simulink model "Verification_Actuator_Primitive"  (R2012b)
settings: Solver=FixedStepDiscrete  StartTime=0.0  StopTime=10.0  FixedStep=0.1  RelTol=1e-3
libraries: sldvlib x7
settings Model: Creator=Kerianne  LastModifiedBy=Kerianne
settings DataIOCC: SaveFormat=Structure
settings OptimizationCC: InlineParams=on

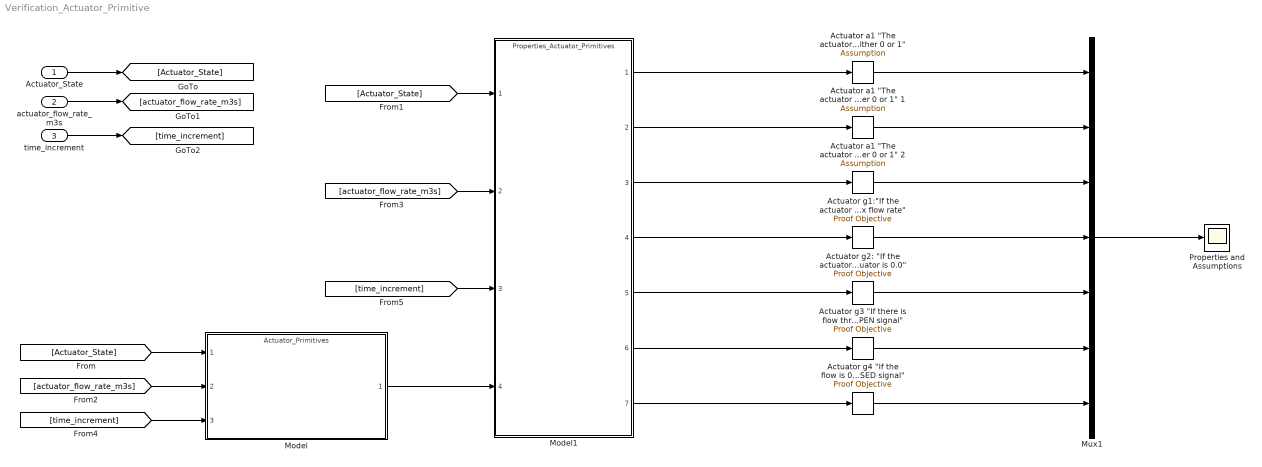
== system Verification_Actuator_Primitive ==
  Actuator_State : Inport  OutDataTypeStr=double
  actuator_flow_rate_m3s : Inport  Port=2  OutDataTypeStr=double
  time_increment : Inport  Port=3  OutDataTypeStr=double
  "Actuator a1 \"The actuator state is either 0 or 1\" " : sldvlib/Objectives and Constraints/Assumption  enabled=on  customAVTBlockType=Assumption  intervals=true  initial=off  dispValues=on  outEnabled=on
      settings: AttributesFormatString=%<intervals>
  "Actuator a1 \"The actuator state is either 0 or 1\" 1" : sldvlib/Objectives and Constraints/Assumption  enabled=on  customAVTBlockType=Assumption  intervals=true  initial=off  dispValues=on  outEnabled=on
      settings: AttributesFormatString=%<intervals>
  "Actuator a1 \"The actuator state is either 0 or 1\" 2" : sldvlib/Objectives and Constraints/Assumption  enabled=on  customAVTBlockType=Assumption  intervals=true  initial=off  dispValues=on  outEnabled=on
      settings: AttributesFormatString=%<intervals>
  "Actuator g1:\"If the actuator is receiving an ON|OPEN signal then the flow through the actuator is the max flow rate\"" : sldvlib/Objectives and Constraints/Proof Objective  enabled=on  customAVTBlockType=Proof Objective  intervals=true  dispValues=on  outEnabled=on  enableStopSim=off
      settings: AttributesFormatString=%<intervals>
  "Actuator g2: \"If the actuator is receiving an OFF|CLOSED signal then the flow rate through the actuator is 0.0\"" : sldvlib/Objectives and Constraints/Proof Objective  enabled=on  customAVTBlockType=Proof Objective  intervals=true  dispValues=on  outEnabled=on  enableStopSim=off
      settings: AttributesFormatString=%<intervals>
  "Actuator g3 \"If there is flow through the actuator, then the actuator is receiving an ON|OPEN signal\"" : sldvlib/Objectives and Constraints/Proof Objective  enabled=on  customAVTBlockType=Proof Objective  intervals=true  dispValues=on  outEnabled=on  enableStopSim=off
      settings: AttributesFormatString=%<intervals>
  "Actuator g4 \"If the flow is 0.0, then the pump is receiving on OFF|CLOSED signal\"" : sldvlib/Objectives and Constraints/Proof Objective  enabled=on  customAVTBlockType=Proof Objective  intervals=true  dispValues=on  outEnabled=on  enableStopSim=off
      settings: AttributesFormatString=%<intervals>
  Model : ModelReference  ModelNameDialog=Actuator_Primitives  SimulationMode=Normal  ModelReferenceVersion=1.26  CopyOfModelName=Actuator_Primitives  DefaultDataLogging=on
  Model1 : ModelReference  ModelNameDialog=Properties_Actuator_Primitives  SimulationMode=Normal  ModelReferenceVersion=1.16  CopyOfModelName=Properties_Actuator_Primitives  DefaultDataLogging=on
  Mux1 : Mux  Inputs=7
  Properties and Assumptions : Scope
  wires:
  Model/1 -> Model1/4
  "Actuator g4 \"If the flow is 0.0, then the pump is receiving on OFF|CLOSED signal\""/1 -> Mux1/7
  "Actuator g1:\"If the actuator is receiving an ON|OPEN signal then the flow through the actuator is the max flow rate\""/1 -> Mux1/4
  Model1/7 -> "Actuator g4 \"If the flow is 0.0, then the pump is receiving on OFF|CLOSED signal\""/1
  Model1/4 -> "Actuator g1:\"If the actuator is receiving an ON|OPEN signal then the flow through the actuator is the max flow rate\""/1
  "Actuator g2: \"If the actuator is receiving an OFF|CLOSED signal then the flow rate through the actuator is 0.0\""/1 -> Mux1/5
  "Actuator g3 \"If there is flow through the actuator, then the actuator is receiving an ON|OPEN signal\""/1 -> Mux1/6
  Model1/5 -> "Actuator g2: \"If the actuator is receiving an OFF|CLOSED signal then the flow rate through the actuator is 0.0\""/1
  Mux1/1 -> Properties and Assumptions/1
  Model1/6 -> "Actuator g3 \"If there is flow through the actuator, then the actuator is receiving an ON|OPEN signal\""/1
  Actuator_State/1 -> [Actuator_State]
  actuator_flow_rate_m3s/1 -> [actuator_flow_rate_m3s]
  time_increment/1 -> [time_increment]
  [time_increment] -> Model/3
  [actuator_flow_rate_m3s] -> Model/2
  [Actuator_State] -> Model/1
  [time_increment] -> Model1/3
  [actuator_flow_rate_m3s] -> Model1/2
  [Actuator_State] -> Model1/1
  Model1/1 -> "Actuator a1 \"The actuator state is either 0 or 1\" "/1
  Model1/2 -> "Actuator a1 \"The actuator state is either 0 or 1\" 1"/1
  Model1/3 -> "Actuator a1 \"The actuator state is either 0 or 1\" 2"/1
  "Actuator a1 \"The actuator state is either 0 or 1\" 2"/1 -> Mux1/3
  "Actuator a1 \"The actuator state is either 0 or 1\" 1"/1 -> Mux1/2
  "Actuator a1 \"The actuator state is either 0 or 1\" "/1 -> Mux1/1
